simulink model "R5_EMB_GENERAL"  (R2024b)
settings: Solver=ode5  StartTime=0.0  StopTime=S  FixedStep=T  RelTol=1e-3  EnableMultiTasking=on
undefined symbols (not defined in the file): Serial_Port, Standard_Devices, T
libraries: easyio x8
settings Model: ModifiedByFormat=C. Gokcek  SimulationMode=external  ExtModeTrigDuration=20480  Creator=C. Gokcek  LastModifiedBy=C. Gokcek
settings SolverCC: AlgebraicLoopSolver=TrustRegion
settings DataIOCC: SaveFormat=Array  SaveOutput=off  SignalLogging=off  DSMLogging=off  SaveTime=off  ReturnWorkspaceOutputs=off
settings OptimizationCC: ReuseModelBlockBuffer=off  ExpressionDepthLimit=2147483647  InitFltsAndDblsToZero=on  EfficientMapNaN2IntZero=off  LifeSpan=inf  SimCompilerOptimization=on
settings DebuggingCC: UnderspecifiedInitializationDetection=Classic  MergeDetectMultiDrivingBlocksExec=none  UnconnectedInputMsg=warning  UnconnectedOutputMsg=warning  UnconnectedLineMsg=warning  AllowSymbolicDim=off  StateNameClashWarn=warning  SFUnexpectedBacktrackingDiag=warning  SFNoUnconditionalDefaultTransitionDiag=warning  SFExecutionAtInitializationDiag=none  ArithmeticOperatorsInVariantConditions=warning
settings HardwareCC: ProdBitPerLong=64  ProdHWDeviceType=Intel->x86-64 (Linux 64)  TargetBitPerLong=64  TargetBitPerPointer=64  TargetIntDivRoundTo=Zero  TargetEndianess=LittleEndian  TargetWordSize=64  TargetHWDeviceType=Intel->x86-64
settings ModelReferenceCC: EnableRefExpFcnMdlSchedulingChecks=on  PropagateSignalLabelsOutOfModel=off
settings SFSimCC: SimUseLocalCustomCode=off  CustomCodeUndefinedFunction=UseInterfaceOnly
settings RTWCC: Description=Simulink Desktop Real-Time  SystemTargetFile=sldrt.tlc  TemplateMakefile=sldrt.tmf  RTWVerbose=off  TLCAssert=on  RTWUseLocalCustomCode=off  RTWCompilerOptimization=on  GPUComputeCapability=3.5  DLArmComputeVersion=19.05
settings CodeAppCC: GenerateComments=off  MaxIdLength=95  SimulinkBlockComments=off
settings SimulinkDesktopRealTimeCC: TargetLibSuffix=_sldrt.a  TargetPreCompLibLocation=C:\Program Files\MATLAB\R2024b\toolbox\sldrt\lib\win64  TargetLangStandard=C89/C90 (ANSI)  ParMdlRefBuildCompliant=on  SupportVariableSizeSignals=off
settings ConfigComp: CovMetricSettings=dw  CovSaveCumulativeToWorkspaceVar=on  CovSaveSingleToWorkspaceVar=on  CovExternalEMLEnable=off  CovSFcnEnable=off

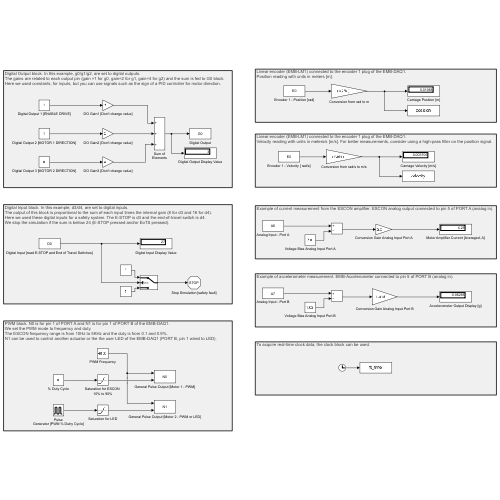
[thumbnail: Simulink's stored preview of the top-level diagram]
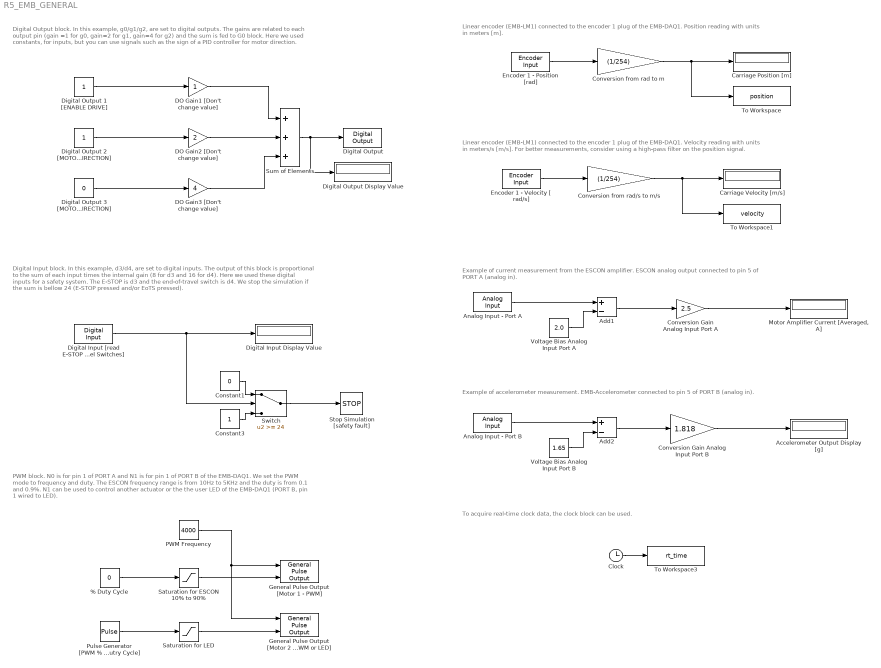
== system R5_EMB_GENERAL ==
  note: Example of current measurement from the ESCON amplifier. ESCON analog output connected to pin 5 of PORT A (analog in).
  note: Example of accelerometer measurement. EMB-Accelerometer connected to pin 5 of PORT B (analog in).
  note: Linear encoder (EMB-LM1) connected to the encoder 1 plug of the EMB-DAQ1.
      | Position reading with units in meters [m].
  note: Linear encoder (EMB-LM1) connected to the encoder 1 plug of the EMB-DAQ1.
      | Velocity reading with units in meters/s [m/s]. For better measurements, consider using a high-pass filter on the position signal.
  note: Digital Output block. In this example, g0/g1/g2, are set to digital outputs.
      | The gains are related to each output pin (gain =1 for g0, gain=2 for g1, gain=4 for g2) and the sum is fed to G0 block.
      | Here we used constants, for inputs, but you can use signals such as the sign of a PID controller for motor direction.
  note: Digital Input block. In this example, d3/d4, are set to digital inputs.
      | The output of this block is proportional to the sum of each input times the internal gain (8 for d3 and 16 for d4).
      | Here we used these digital inputs for a safety system. The E-STOP is d3 and the end-of-travel switch is d4.
      | We stop the simulation if the sum is bellow 24 (E-STOP pressed and/or EoTS pressed).
  note: PWM block. N0 is for pin 1 of PORT A and N1 is for pin 1 of PORT B of the EMB-DAQ1.
      | We set the PWM mode to frequency and duty.
      | The ESCON frequency range is from 10Hz to 5KHz and the duty is from 0.1 and 0.9%.
      | N1 can be used to control another actuator or the the user LED of the EMB-DAQ1 (PORT B, pin 1 wired to LED).
  note: To acquire real-time clock data, the clock block can be used.
  % Duty Cycle : Constant  Value=0
  Accelerometer Output Display [g] : Display
  Add1 : Sum  Inputs=+-
  Add2 : Sum  Inputs=+-
  Analog Input - Port A : easyio/Analog Input  SampleTime=T  MaxMissedTicks=10  ShowMissedTicks=0  YieldWhenWaiting=0  DrvName=Standard_Devices/Serial_Port  DrvAddress=6  DrvOptions=[460800 8 0 0 0 0 0 0]  PacketSize=8  DataTypes='double'  ShowReady=0  ShowError=0  PacketID=1  ByteOrder=1  ShowTimestamp=0  CfgPrm=A6  PrmCfg=unipolar  ResVar=0  VarRes=0
      settings: SourceProductName=Easyio
  Analog Input - Port B : easyio/Analog Input  SampleTime=T  MaxMissedTicks=10  ShowMissedTicks=0  YieldWhenWaiting=0  DrvName=Standard_Devices/Serial_Port  DrvAddress=6  DrvOptions=[460800 8 0 0 0 0 0 0]  PacketSize=8  DataTypes='double'  ShowReady=0  ShowError=0  PacketID=1  ByteOrder=1  ShowTimestamp=0  CfgPrm=A7  PrmCfg=unipolar  ResVar=0  VarRes=0
      settings: SourceProductName=Easyio
  Carriage Position [m] : Display
  Carriage Velocity [m/s] : Display
  Clock : Clock
  Constant1 : Constant  Value=0
  Constant3 : Constant
  Conversion Gain Analog Input Port A : Gain  Gain=2.5
  Conversion Gain Analog Input Port B : Gain  Gain=1.818
  Conversion from rad to m : Gain  Gain=(1/254)
  Conversion from rad/s to m/s : Gain  Gain=(1/254)
  DO Gain1 [Don't change value] : Gain
  DO Gain2 [Don't change value] : Gain  Gain=2
  DO Gain3 [Don't change value] : Gain  Gain=4
  Digital Input Display Value : Display
  Digital Input [read E-STOP and End of Travel Switches] : easyio/Digital Input  SampleTime=T  MaxMissedTicks=10  ShowMissedTicks=0  YieldWhenWaiting=0  DrvName=Standard_Devices/Serial_Port  DrvAddress=6  DrvOptions=[460800 8 0 0 0 0 0 0]  PacketSize=8  DataTypes='double'  ShowReady=0  ShowError=0  PacketID=1  ByteOrder=1  ShowTimestamp=0  CfgPrm=D0  PrmCfg=18  ResVar=0  VarRes=0  d7=off  d6=off  d5=off  d4=on  d3=on  d2=off  d1=off  d0=off
      settings: SourceProductName=Easyio
  Digital Output : easyio/Digital Output  SampleTime=T  MaxMissedTicks=10  ShowMissedTicks=0  YieldWhenWaiting=0  DrvName=Standard_Devices/Serial_Port  DrvAddress=6  DrvOptions=[460800 8 0 0 0 0 0 0]  PacketSize=8  DataTypes='double'  ShowReady=0  ShowError=0  PacketID=1  ByteOrder=1  InitialValue=0  FinalValue=0  CfgPrm=G0  PrmCfg=F8  ResVar=0  VarRes=0  d7=off  d6=off  d5=off  d4=off  d3=off  d2=on  d1=on  d0=on
      settings: SourceProductName=Easyio
  Digital Output 1 [ENABLE DRIVE] : Constant
  Digital Output 2 [MOTOR 1 DIRECTION] : Constant
  Digital Output 3 [MOTOR 2 DIRECTION] : Constant  Value=0
  Digital Output Display Value : Display
  Encoder 1 - Position [rad] : easyio/Encoder Input  SampleTime=T  MaxMissedTicks=10  ShowMissedTicks=0  YieldWhenWaiting=0  DrvName=Standard_Devices/Serial_Port  DrvAddress=6  DrvOptions=[460800 8 0 0 0 0 0 0]  PacketSize=8  DataTypes='double'  ShowReady=0  ShowError=0  PacketID=1  ByteOrder=1  ShowTimestamp=0  CfgPrm=E0  PrmCfg=position  ResVar=0  VarRes=2000
      settings: SourceProductName=Easyio
  Encoder 1 - Velocity [ rad/s] : easyio/Encoder Input  SampleTime=T  MaxMissedTicks=10  ShowMissedTicks=0  YieldWhenWaiting=0  DrvName=Standard_Devices/Serial_Port  DrvAddress=6  DrvOptions=[460800 8 0 0 0 0 0 0]  PacketSize=8  DataTypes='double'  ShowReady=0  ShowError=0  PacketID=1  ByteOrder=1  ShowTimestamp=0  CfgPrm=E0  PrmCfg=velocity  ResVar=0  VarRes=2000
      settings: SourceProductName=Easyio
  General Pulse Output [Motor 1 - PWM] : easyio/General Pulse Output  SampleTime=T  MaxMissedTicks=10  ShowMissedTicks=0  YieldWhenWaiting=0  DrvName=Standard_Devices/Serial_Port  DrvAddress=6  DrvOptions=[460800 8 0 0 0 0 0 0]  PacketSize=16  DataTypes={'double','double'}  ShowReady=0  ShowError=0  PacketID=1  ByteOrder=1  InitialValue=[0 0]  FinalValue=[0 0]  CfgPrm=N0  PrmCfg=frequency and duty  ResVar=449.8360 Hz - 115156.25 Hz  VarRes=64
      settings: SourceProductName=Easyio
  General Pulse Output [Motor 2 - PWM or LED] : easyio/General Pulse Output  SampleTime=T  MaxMissedTicks=10  ShowMissedTicks=0  YieldWhenWaiting=0  DrvName=Standard_Devices/Serial_Port  DrvAddress=6  DrvOptions=[460800 8 0 0 0 0 0 0]  PacketSize=16  DataTypes={'double','double'}  ShowReady=0  ShowError=0  PacketID=1  ByteOrder=1  InitialValue=[0 0]  FinalValue=[0 0]  CfgPrm=N1  PrmCfg=frequency and duty  ResVar=449.8360 Hz - 115156.25 Hz  VarRes=64
      settings: SourceProductName=Easyio
  "Motor Amplifier Current [Averaged, A]" : Display
  PWM Frequency : Constant  Value=4000
  Pulse Generator [PWM % Dutry Cycle] : DiscretePulseGenerator  PulseType=Time based  Period=0.4  PulseWidth=50
  Saturation for ESCON 10% to 90% : Saturate  UpperLimit=0.9  LowerLimit=0.1
  Saturation for LED : Saturate  UpperLimit=1  LowerLimit=0
  Stop Simulation [safety fault] : Stop
  Sum of Elements : Sum  Inputs=+++
  Switch : Switch  Threshold=24  SaturateOnIntegerOverflow=off  InputSameDT=off
  To Workspace : ToWorkspace  VariableName=position  SampleTime=-1
  To Workspace1 : ToWorkspace  VariableName=velocity  SampleTime=-1
  To Workspace3 : ToWorkspace  VariableName=rt_time  SampleTime=-1
  Voltage Bias Analog Input Port A : Constant  Value=2.0
  Voltage Bias Analog Input Port B : Constant  Value=1.65
  wires:
  Encoder 1 - Position [rad]/1 -> Conversion from rad to m/1
  PWM Frequency/1 -> General Pulse Output [Motor 1 - PWM]/1, General Pulse Output [Motor 2 - PWM or LED]/1
  Digital Output 1 [ENABLE DRIVE]/1 -> DO Gain1 [Don't change value]/1
  Sum of Elements/1 -> Digital Output/1, Digital Output Display Value/1
  DO Gain2 [Don't change value]/1 -> Sum of Elements/2
  DO Gain1 [Don't change value]/1 -> Sum of Elements/1
  Saturation for LED/1 -> General Pulse Output [Motor 2 - PWM or LED]/2
  Pulse Generator [PWM % Dutry Cycle]/1 -> Saturation for LED/1
  Digital Output 3 [MOTOR 2 DIRECTION]/1 -> DO Gain3 [Don't change value]/1
  DO Gain3 [Don't change value]/1 -> Sum of Elements/3
  Digital Input [read E-STOP and End of Travel Switches]/1 -> Switch/2, Digital Input Display Value/1
  Switch/1 -> Stop Simulation [safety fault]/1
  Constant1/1 -> Switch/1
  Constant3/1 -> Switch/3
  Voltage Bias Analog Input Port A/1 -> Add1/2
  Analog Input - Port A/1 -> Add1/1
  Add1/1 -> Conversion Gain Analog Input Port A/1
  Voltage Bias Analog Input Port B/1 -> Add2/2
  Add2/1 -> Conversion Gain Analog Input Port B/1
  Analog Input - Port B/1 -> Add2/1
  Conversion Gain Analog Input Port B/1 -> Accelerometer Output Display [g]/1
  Conversion Gain Analog Input Port A/1 -> "Motor Amplifier Current [Averaged, A]"/1
  Conversion from rad to m/1 -> To Workspace/1, Carriage Position [m]/1
  Conversion from rad/s to m/s/1 -> To Workspace1/1, Carriage Velocity [m/s]/1
  Encoder 1 - Velocity [ rad/s]/1 -> Conversion from rad/s to m/s/1
  Clock/1 -> To Workspace3/1
  Digital Output 2 [MOTOR 1 DIRECTION]/1 -> DO Gain2 [Don't change value]/1
  % Duty Cycle/1 -> Saturation for ESCON 10% to 90%/1
  Saturation for ESCON 10% to 90%/1 -> General Pulse Output [Motor 1 - PWM]/2
